simulink model "simphone"  (R2017b)
settings: Solver=FixedStepDiscrete  StartTime=0.0  StopTime=10.0  RelTol=1e-3
libraries: simulink x1
settings Model: DataTypeOverride=Off  Creator=Daniel Yang  LastModifiedBy=Daniel Yang
settings DataIOCC: SaveOutput=off  SaveTime=off
settings OptimizationCC: BlockReduction=off  ConditionallyExecuteInputs=off  DefaultParameterBehavior=Inlined
settings DebuggingCC: AlgebraicLoopMsg=error  SingleTaskRateTransMsg=error
settings HardwareCC: ProdBitPerPointer=32  ProdBitPerSizeT=32  ProdBitPerPtrDiffT=32  ProdLargestAtomicFloat=None  ProdIntDivRoundTo=Undefined  ProdEndianess=Unspecified  ProdWordSize=32  ProdHWDeviceType=ASIC/FPGA->ASIC/FPGA  TargetBitPerPointer=64  TargetBitPerSizeT=64  TargetBitPerPtrDiffT=64  TargetLongLongMode=on  TargetIntDivRoundTo=Zero  TargetEndianess=LittleEndian  TargetWordSize=64  TargetHWDeviceType=Custom Processor->MATLAB Host Computer  ProdEqTarget=off

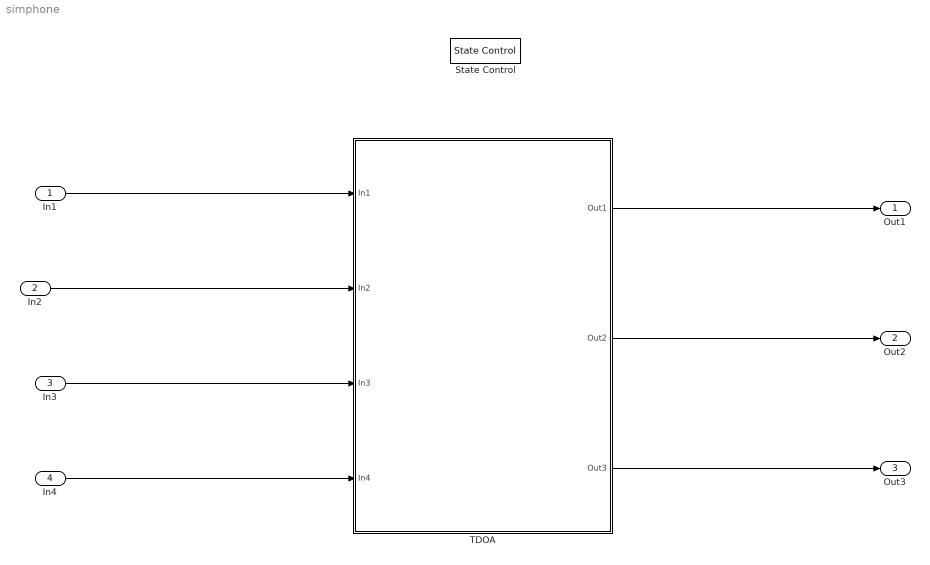
== system simphone ==
  In1 : Inport  OutDataTypeStr=boolean
  In2 : Inport  Port=2  OutDataTypeStr=boolean
  In3 : Inport  Port=3  OutDataTypeStr=boolean
  In4 : Inport  Port=4  OutDataTypeStr=boolean
  State Control : StateControl  StateControl=Synchronous
  TDOA : Subsystem
  Out1 : Outport
  Out2 : Outport  Port=2
  Out3 : Outport  Port=3
  wires:
  In1/1 -> TDOA/1(In1)
  In2/1 -> TDOA/2(In2)
  In3/1 -> TDOA/3(In3)
  In4/1 -> TDOA/4(In4)
  TDOA/1(Out1) -> Out1/1
  TDOA/3(Out3) -> Out3/1
  TDOA/2(Out2) -> Out2/1

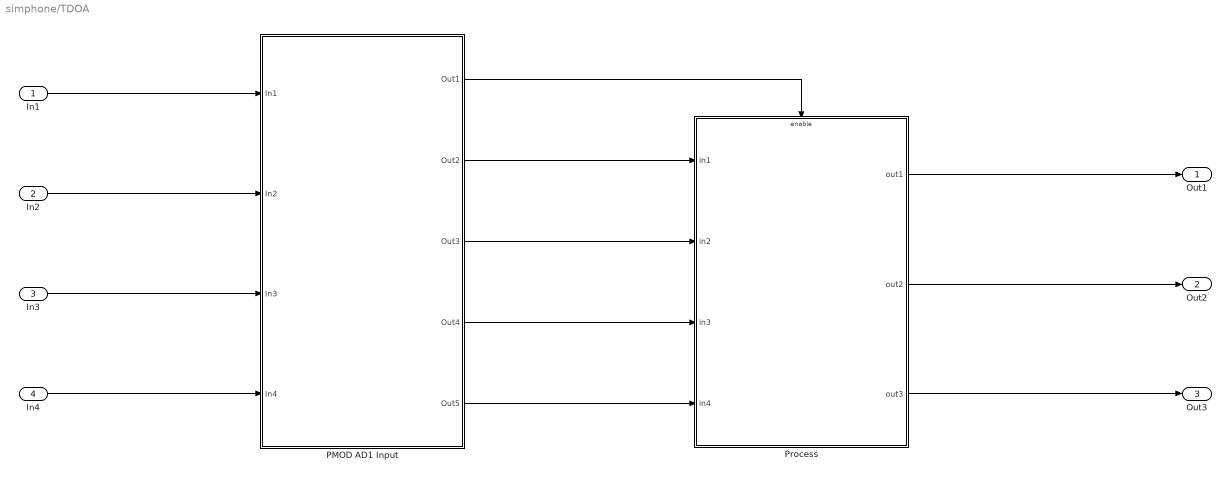
== system simphone/TDOA ==
  In1 : Inport
  In2 : Inport  Port=2
  In3 : Inport  Port=3
  In4 : Inport  Port=4
  PMOD AD1 Input : Subsystem
  Process : Subsystem  TreatAsAtomicUnit=on
  Out1 : Outport
  Out2 : Outport  Port=2
  Out3 : Outport  Port=3
  wires:
  Process/2(out2) -> Out2/1
  Process/1(out1) -> Out1/1
  Process/3(out3) -> Out3/1
  In1/1 -> PMOD AD1 Input/1(In1)
  In2/1 -> PMOD AD1 Input/2(In2)
  In3/1 -> PMOD AD1 Input/3(In3)
  In4/1 -> PMOD AD1 Input/4(In4)
  PMOD AD1 Input/1(Out1) -> Process/Enable
  PMOD AD1 Input/2(Out2) -> Process/1(in1)
  PMOD AD1 Input/3(Out3) -> Process/2(in2)
  PMOD AD1 Input/4(Out4) -> Process/3(in3)
  PMOD AD1 Input/5(Out5) -> Process/4(in4)

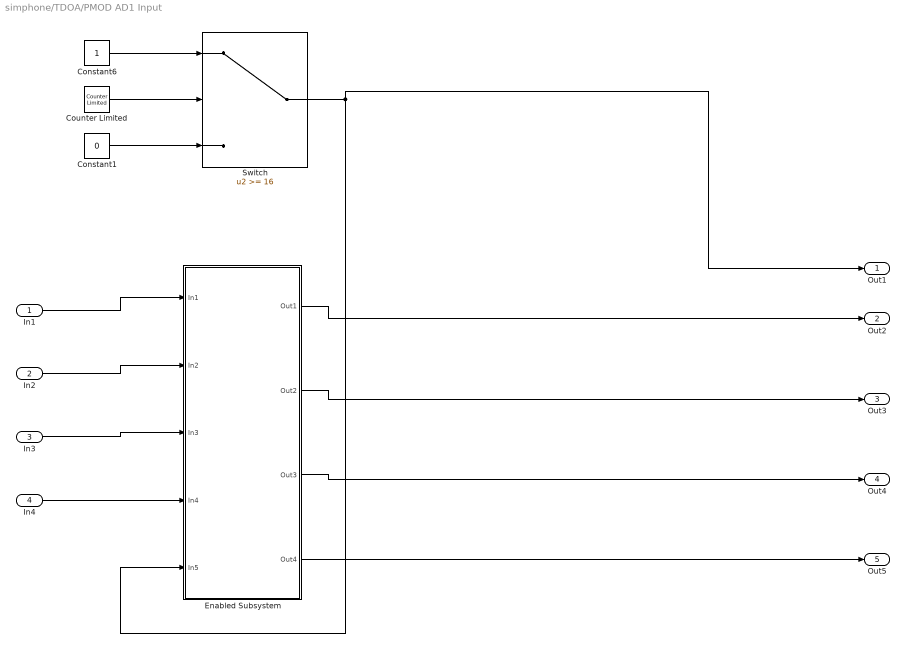
== system simphone/TDOA/PMOD AD1 Input ==
  In1 : Inport
  In2 : Inport  Port=2
  In3 : Inport  Port=3
  In4 : Inport  Port=4
  Constant1 : Constant  Value=0  OutDataTypeStr=boolean
  Constant6 : Constant  OutDataTypeStr=boolean
  Counter Limited : simulink/Sources/Counter Limited  uplimit=15  tsamp=-1
  Enabled Subsystem : Subsystem  TreatAsAtomicUnit=on
  Switch : Switch  Threshold=16
  Out1 : Outport
  Out2 : Outport  Port=2
  Out3 : Outport  Port=3
  Out4 : Outport  Port=4
  Out5 : Outport  Port=5
  wires:
  Enabled Subsystem/2(Out2) -> Out3/1
  Switch/1 -> Enabled Subsystem/5(In5), Out1/1
  In4/1 -> Enabled Subsystem/4(In4)
  In2/1 -> Enabled Subsystem/2(In2)
  Enabled Subsystem/4(Out4) -> Out5/1
  Constant1/1 -> Switch/3
  Counter Limited/1 -> Switch/2
  Constant6/1 -> Switch/1
  Enabled Subsystem/3(Out3) -> Out4/1
  In1/1 -> Enabled Subsystem/1(In1)
  Enabled Subsystem/1(Out1) -> Out2/1
  In3/1 -> Enabled Subsystem/3(In3)

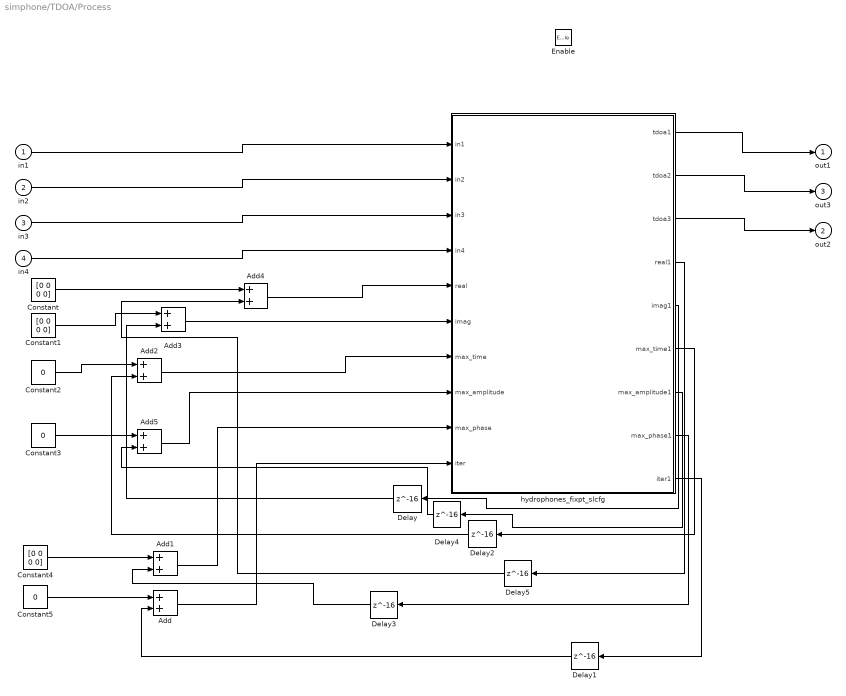
== system simphone/TDOA/Process ==
  in1 : Inport
  in2 : Inport  Port=2
  in3 : Inport  Port=3
  in4 : Inport  Port=4
  Enable : EnablePort
  Add : Sum  OutDataTypeStr=fixdt(0,24,0)
  Add1 : Sum  OutDataTypeStr=fixdt(0,16,15)
  Add2 : Sum  OutDataTypeStr=fixdt(0,26,0)
  Add3 : Sum  OutDataTypeStr=fixdt(1,16,3)
  Add4 : Sum  OutDataTypeStr=fixdt(1,16,3)
  Add5 : Sum  OutDataTypeStr=fixdt(1,16,8)
  Constant : Constant  Value=[0 0 0 0]  OutDataTypeStr=fixdt(1,16,3)
  Constant1 : Constant  Value=[0 0 0 0]  OutDataTypeStr=fixdt(1,16,3)
  Constant2 : Constant  Value=0  OutDataTypeStr=fixdt(0,26,0)
  Constant3 : Constant  Value=0  OutDataTypeStr=fixdt(1,16,8)
  Constant4 : Constant  Value=[0 0 0 0]  OutDataTypeStr=fixdt(0,16,15)
  Constant5 : Constant  Value=0  OutDataTypeStr=fixdt(0,24,0)
  Delay{,1..5} (6 alike) : Delay  DelayLength=16
  hydrophones_fixpt_slcfg : MATLAB Function  TreatAsAtomicUnit=on
  out1 : Outport
  out2 : Outport  Port=2
  out3 : Outport  Port=3
  wires:
  in3/1 -> hydrophones_fixpt_slcfg/3(in3)
  in2/1 -> hydrophones_fixpt_slcfg/2(in2)
  in1/1 -> hydrophones_fixpt_slcfg/1(in1)
  in4/1 -> hydrophones_fixpt_slcfg/4(in4)
  hydrophones_fixpt_slcfg/4(real1) -> Delay5/1
  hydrophones_fixpt_slcfg/5(imag1) -> Delay/1
  hydrophones_fixpt_slcfg/6(max_time1) -> Delay2/1
  hydrophones_fixpt_slcfg/7(max_amplitude1) -> Delay4/1
  hydrophones_fixpt_slcfg/8(max_phase1) -> Delay3/1
  hydrophones_fixpt_slcfg/9(iter1) -> Delay1/1
  hydrophones_fixpt_slcfg/1(tdoa1) -> out1/1
  hydrophones_fixpt_slcfg/2(tdoa2) -> out3/1
  hydrophones_fixpt_slcfg/3(tdoa3) -> out2/1
  Add/1 -> hydrophones_fixpt_slcfg/10(iter)
  Delay1/1 -> Add/2
  Constant5/1 -> Add/1
  Constant4/1 -> Add1/1
  Delay3/1 -> Add1/2
  Add1/1 -> hydrophones_fixpt_slcfg/9(max_phase)
  Constant2/1 -> Add2/1
  Delay2/1 -> Add2/2
  Add2/1 -> hydrophones_fixpt_slcfg/7(max_time)
  Delay/1 -> Add3/2
  Constant1/1 -> Add3/1
  Add3/1 -> hydrophones_fixpt_slcfg/6(imag)
  Delay5/1 -> Add4/2
  Constant/1 -> Add4/1
  Add4/1 -> hydrophones_fixpt_slcfg/5(real)
  Constant3/1 -> Add5/1
  Delay4/1 -> Add5/2
  Add5/1 -> hydrophones_fixpt_slcfg/8(max_amplitude)

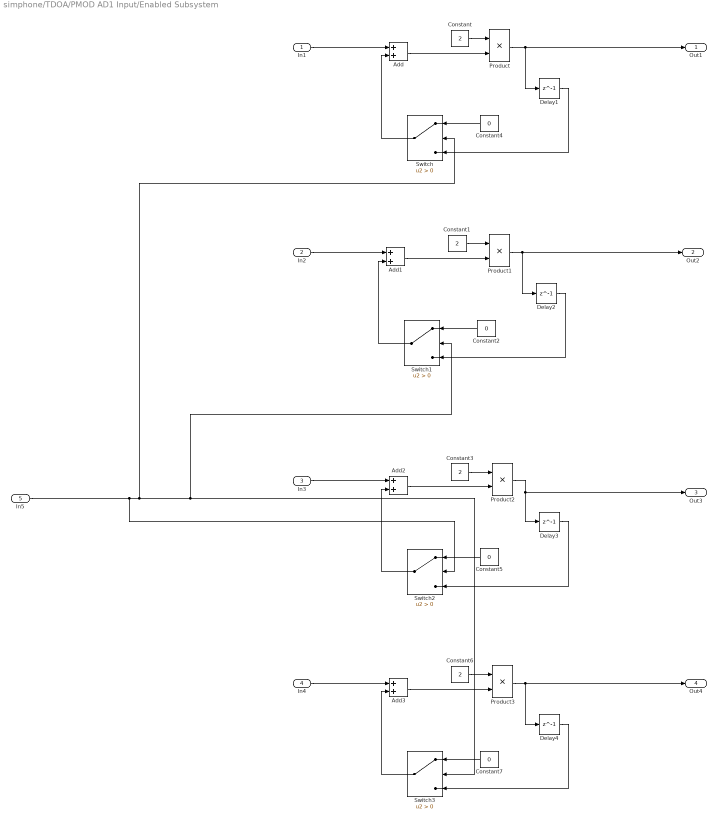
== system simphone/TDOA/PMOD AD1 Input/Enabled Subsystem ==
  In1 : Inport
  In2 : Inport  Port=2
  In3 : Inport  Port=3
  In4 : Inport  Port=4
  In5 : Inport  Port=5
  Add{,1..3} (4 alike) : Sum
  Constant : Constant  Value=2
  Constant1 : Constant  Value=2  OutDataTypeStr=fixdt(1,12,9)
  Constant{2,4..5,7} (4 alike) : Constant  Value=0
  Constant3 : Constant  Value=2
  Constant6 : Constant  Value=2
  Delay{1..4} (4 alike) : Delay  DelayLength=1  InitialCondition=0
  Product{,1..3} (4 alike) : Product  OutDataTypeStr=fixdt(0,12,0)
  Switch{,1..3} (4 alike) : Switch  Criteria=u2 > Threshold
  Out1 : Outport
  Out2 : Outport  Port=2
  Out3 : Outport  Port=3
  Out4 : Outport  Port=4
  wires:
  Constant/1 -> Product/1
  Product/1 -> Out1/1, Delay1/1
  Add/1 -> Product/2
  In1/1 -> Add/1
  Switch/1 -> Add/2
  Constant4/1 -> Switch/1
  Delay1/1 -> Switch/3
  In5/1 -> Switch2/2, Switch/2, Switch1/2, Switch3/2
  In2/1 -> Add1/1
  Switch1/1 -> Add1/2
  Constant1/1 -> Product1/1
  Product1/1 -> Out2/1, Delay2/1
  Constant2/1 -> Switch1/1
  Add1/1 -> Product1/2
  Delay2/1 -> Switch1/3
  In3/1 -> Add2/1
  Switch2/1 -> Add2/2
  Constant3/1 -> Product2/1
  Product2/1 -> Out3/1, Delay3/1
  Constant5/1 -> Switch2/1
  Add2/1 -> Product2/2
  Delay3/1 -> Switch2/3
  In4/1 -> Add3/1
  Switch3/1 -> Add3/2
  Constant6/1 -> Product3/1
  Product3/1 -> Out4/1, Delay4/1
  Constant7/1 -> Switch3/1
  Add3/1 -> Product3/2
  Delay4/1 -> Switch3/3

== matlab function simphone/TDOA/Process/hydrophones_fixpt_slcfg ==
  data: in1 input fixdt('ufix12') size=[1 1 ]; in2 input fixdt('ufix12') size=[1 1 ]; in3 input fixdt('ufix12') size=[1 1 ]; in4 input fixdt('ufix12') size=[1 1 ]; tdoa1 output; tdoa2 output; tdoa3 output; real input; imag input; max_time input; max_amplitude input; max_phase input; iter input; real1 output; imag1 output; max_time1 output; max_amplitude1 output; max_phase1 output; iter1 output
%%%%%%%%%%%%%%%%%%%%%%%%%%%%%%%%%%%%%%%%%%%%%%%%%%%%%%%%%%%%%%%%%%%%%%%%%%%%
%                                                                          %
%           Generated by MATLAB 9.3 and Fixed-Point Designer 6.0           %
%                                                                          %
%%%%%%%%%%%%%%%%%%%%%%%%%%%%%%%%%%%%%%%%%%%%%%%%%%%%%%%%%%%%%%%%%%%%%%%%%%%%
%#codegen
function [tdoa1,tdoa2,tdoa3,real1,imag1,max_time1,max_amplitude1,max_phase1,iter1]=hydrophones_fixpt(in1,in2,in3,in4,real,imag,max_time,max_amplitude,max_phase,iter)
  fm = get_fimath();

  alpha = fi(.99, 0, 16, 16, fm);
  beta = fi(.01, 0, 16, 22, fm);
  out = fi(zeros(3), 1, 16, 13, fm);
  frequency=fi(25000, 0, 15, 0, fm);
  sine_wave_size = fi(200, 0, 8, 0, fm);
  sampling_rate = fi(200000, 0, 18, 0, fm);
  window = fi(1996000, 0, 21, 0, fm);
  threshold = fi(0, 0, 1, 0, fm);
  
  in = fi([fi(in1, 0, 12, 0, fm) in2 in3 in4], 0, 12, 0, fm);
  
  time = fi(fi_div(iter * fi(1000000, 0, 24, 0, fm), sampling_rate), 0, 26, 0, fm);
  
  microrevs = fi(mod((frequency * time),fi(1000000, 0, 20, 0, fm)), 0, 20, 0, fm);
  wave_idx = fi(microrevs * sine_wave_size*fi(1/1000000, 0, 16, 35, fm), 0, 8, 0, fm);
      for c=1:4 
         real(c) = real(c) * alpha + in(c) * sin(wave_idx) * beta;
         imag(c) = fi_signed(imag(c) * alpha) - in(c) * cos(wave_idx) * beta;
      end

      if (time > window) 
         if time < max_time
             %F2F: No information found for converting the following block of code
             %F2F: Start block
             max_time(:) = 0;
             %F2F: End block
         end
         min_amplitude = fi(100, 0, 16, 9, fm);

         for c=1:4 
            amplitude = fi(real(c) * real(c) + imag(c) * imag(c), 0, 32, 4, fm);
            if amplitude < min_amplitude 
                min_amplitude(:) = amplitude;
            end
         end

         if (min_amplitude > max_amplitude) 
           max_amplitude(:) = min_amplitude;
           max_time(:) = time;
           for c = 1:4
             y = fi(abs(imag(c)), 0, 16, 5, fm);
             x = fi(abs(real(c)), 0, 16, 6, fm);
             max_phase(c) = atan2(y, x);
           end
         end
         if time - max_time >= window && max_amplitude >= threshold 
            base_phase = fi(max_phase(1), 0, 16, 15, fm);
            for c = 2:4 
              phase_shift = fi(fi_signed(max_phase(c)) - fi_signed(base_phase), 1, 16, 15, fm);

              if phase_shift < fi(-pi, 1, 16, 13, fm)
                  %F2F: No information found for converting the following block of code
                  %F2F: Start block
                  phase_shift(:) = phase_shift+ fi(2 * pi, 0, 16, 13, fm);
                  %F2F: End block
              end
              if phase_shift >= fi(pi, 0, 16, 14, fm)
                  %F2F: No information found for converting the following block of code
                  %F2F: Start block
                  phase_shift(:) = phase_shift - fi(2 * pi, 0, 16, 13, fm);
                  %F2F: End block
              end
              time_diff = fi(fi_div(phase_shift, (fi(2 * pi, 0, 16, 13, fm) * frequency)) * fi(1000000, 0, 20, 0, fm), 1, 16, 13, fm);
              out(c-1)=time_diff;
            end

            max_amplitude(:) = -1;
            max_time(:) = time;

            for c = 1:4
              real(c) = 0;
              imag(c) = 0;
            end
         end
      end
      iter(:)=iter+fi(1, 0, 1, 0, fm);
      tdoa1=fi(out(1), 1, 8, 6, fm);
      tdoa2=fi(out(2), 1, 8, 6, fm);
      tdoa3=fi(out(3), 1, 8, 6, fm);
      real1= fi(real, 1, 16, 4, fm);
      imag1= fi(imag, 1, 16, 4, fm);
      max_time1= fi(max_time, 0, 26, 0, fm);
      max_amplitude1= fi(max_amplitude, 1, 16, 8, fm);
      max_phase1= fi(max_phase, 0, 16, 15, fm);
      iter1= fi(iter, 0, 24, 0, fm);
end



function ntype = divideType(a,b)
    coder.inline( 'always' );
    nt1 = numerictype( a );
    nt2 = numerictype( b );
    maxFL = max( [ min( nt1.WordLength, nt1.FractionLength ), min( nt2.WordLength, nt2.FractionLength ) ] );
    FL = max( maxFL, 24 );
    extraBits = (FL - maxFL);
    WL = nt1.WordLength + nt2.WordLength;
    WL = min( WL, 124 );
    if (WL + extraBits)<64
        ntype = numerictype( nt1.Signed || nt2.Signed, WL + extraBits, FL );
    else
        ntype = numerictype( nt1.Signed || nt2.Signed, WL, FL );
    end
end


function c = fi_div(a,b)
    coder.inline( 'always' );
    if isfi( a ) && isfi( b ) && isscalar( b )
        a1 = fi( a, 'RoundMode', 'fix' );
        b1 = fi( b, 'RoundMode', 'fix' );
        c1 = divide( divideType( a1, b1 ), a1, b1 );
        c = fi( c1, numerictype( c1 ), fimath( a ) );
    else
        c = a/b;
    end
end


function y = fi_signed(a)
    coder.inline( 'always' );
    if isfi( a ) && ~(issigned( a ))
        nt = numerictype( a );
        new_nt = numerictype( 1, nt.WordLength + 1, nt.FractionLength );
        y = fi( a, new_nt, fimath( a ) );
    else
        y = a;
    end
end

function fm = get_fimath()
	fm = fimath('RoundingMethod', 'Floor',...
	     'OverflowAction', 'Wrap',...
	     'ProductMode','FullPrecision',...
	     'MaxProductWordLength', 128,...
	     'SumMode','FullPrecision',...
	     'MaxSumWordLength', 128);
end
